simulink model "Copy_of_Qrotor_sim2"  (R2016a)
settings: Solver=ode4  StartTime=0.0  StopTime=T  FixedStep=0.001  RelTol=1e-3
values from neighbouring files (symbols this model uses):
  g = 9.81    [Sim_params.m]
  Ixx = 0.002100    (= 0.0021)    [Drone_params.m]
  Iyy = 0.002417    [Drone_params.m]
  Izz = 0.004633    [Drone_params.m]
  k_learn = 0.000001    (= 1e-06)    [Control_params.m]
  Ki = 3    [Control_params.m]
  KM_1 = KM_GENERAL    (= 0.00509)    [Drone_params.m]
  KM_2 = KM_GENERAL    (= 0.00509)    [Drone_params.m]
  KM_3 = KM_GENERAL    (= 0.00509)    [Drone_params.m]
  KM_4 = KM_GENERAL    (= 0.00509)    [Drone_params.m]
  KM_GENERAL = 0.00509    [Drone_params.m]
  KM_T_1 = KM_T_GENERAL    (= 5e-06)    [Drone_params.m]
  KM_T_2 = KM_T_GENERAL    (= 5e-06)    [Drone_params.m]
  KM_T_3 = KM_T_GENERAL    (= 5e-06)    [Drone_params.m]
  KM_T_4 = KM_T_GENERAL    (= 5e-06)    [Drone_params.m]
  KM_T_GENERAL = 0.000005    (= 5e-06)    [Drone_params.m]
  Kp = Ixx * Ki    [Control_params.m]
  KpP = 5    [Control_params.m]
  m = 0.475    [Drone_params.m]
  n_freq = 0.5    [Sim_params.m]
  PWM_CUT = 1000    [Drone_params.m]
  Tau_1 = Tau    (= 0.1)    [Drone_params.m]
  Tau_2 = Tau    (= 0.1)    [Drone_params.m]
  Tau_3 = Tau    (= 0.1)    [Drone_params.m]
  Tau_4 = Tau    (= 0.1)    [Drone_params.m]
  wnd_amp_p = .1    (= 0.1)    [Wind_params.m]
  wnd_amp_q = 0    [Wind_params.m]
  wnd_amp_r = 0    [Wind_params.m]
  wnd_amp_x = .1    (= 0.1)    [Wind_params.m]
  wnd_amp_y = .1    (= 0.1)    [Wind_params.m]
  wnd_amp_z = .1    (= 0.1)    [Wind_params.m]
  wnd_end_p = 20    [Wind_params.m]
  wnd_end_q = 15    [Wind_params.m]
  wnd_end_r = 15    [Wind_params.m]
  wnd_end_x = 44    [Wind_params.m]
  wnd_end_y = 31    [Wind_params.m]
  wnd_end_z = 49    [Wind_params.m]
  wnd_pqr_enable = 0    [Sim_params.m]
  wnd_ramp_p = 2*pi    (= 6.28318530718)    [Wind_params.m]
  wnd_ramp_q = 0.2    [Wind_params.m]
  wnd_ramp_r = 0.2    [Wind_params.m]
  wnd_ramp_x = .3    (= 0.3)    [Wind_params.m]
  wnd_ramp_y = .3    (= 0.3)    [Wind_params.m]
  wnd_ramp_z = .3    (= 0.3)    [Wind_params.m]
  wnd_start_p = 2    [Wind_params.m]
  wnd_start_q = 2    [Wind_params.m]
  wnd_start_r = 2    [Wind_params.m]
  wnd_start_x = 8    [Wind_params.m]
  wnd_start_y = 3    [Wind_params.m]
  wnd_start_z = 11    [Wind_params.m]
  wnd_xyz_enable = 0    [Sim_params.m]
  X_length = 0.155    [Drone_params.m]
  Y_length = 0.200    (= 0.2)    [Drone_params.m]
undefined symbols (not defined in the file or in its folder): X, Y, Z
libraries: simulink x12, sm_lib x10, nesl_utility x10
(part 2 of 2)

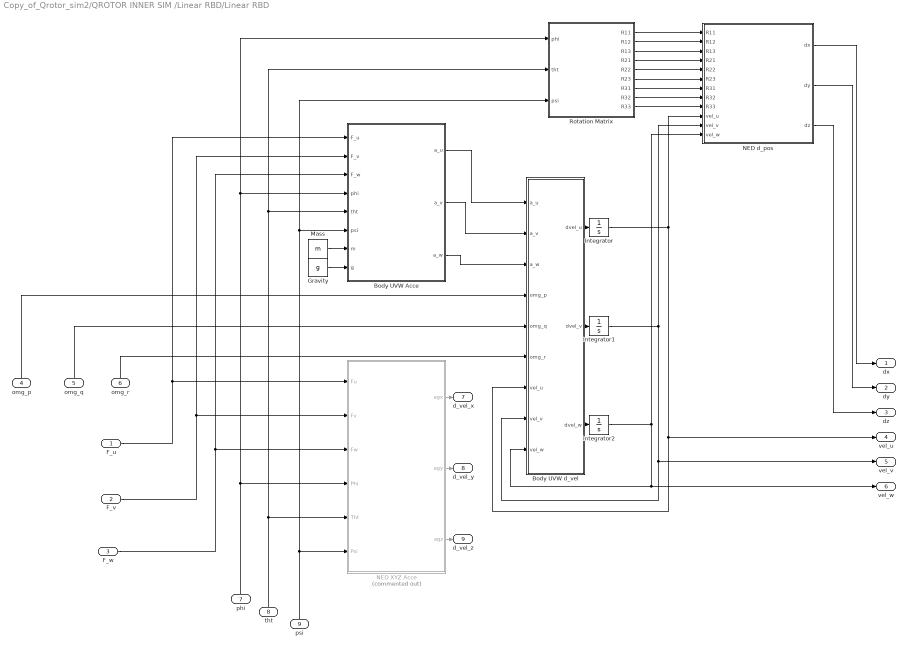
== system Copy_of_Qrotor_sim2/QROTOR INNER SIM /Linear RBD/Linear RBD ==
  F_u : Inport
  F_v : Inport  Port=2
  F_w : Inport  Port=3
  omg_p : Inport  Port=4
  omg_q : Inport  Port=5
  omg_r : Inport  Port=6
  phi : Inport  Port=7
  tht : Inport  Port=8
  psi : Inport  Port=9
  Body UVW Acce : MATLAB Function  TreatAsAtomicUnit=on
  Body UVW d_vel : MATLAB Function  TreatAsAtomicUnit=on
  Gravity : Constant  Value=g
  Integrator : Integrator
  Integrator1 : Integrator
  Integrator2 : Integrator
  Mass : Constant  Value=m
  NED XYZ Acce : Subsystem  Commented=on
  NED d_pos : MATLAB Function  TreatAsAtomicUnit=on
  Rotation Matrix : MATLAB Function  TreatAsAtomicUnit=on
  dx : Outport
  dy : Outport  Port=2
  dz : Outport  Port=3
  vel_u : Outport  Port=4
  vel_v : Outport  Port=5
  vel_w : Outport  Port=6
  d_vel_x : Outport  Port=7
  d_vel_y : Outport  Port=8
  "d_vel_z " : Outport  Port=9
  wires:
  NED d_pos/2(dy) -> dy/1
  Rotation Matrix/5(R22) -> NED d_pos/5(R22)
  NED d_pos/1(dx) -> dx/1
  F_v/1 -> Body UVW Acce/2(F_v), NED XYZ Acce/2(Fv)
  Mass/1 -> Body UVW Acce/7(m)
  Rotation Matrix/1(R11) -> NED d_pos/1(R11)
  Rotation Matrix/9(R33) -> NED d_pos/9(R33)
  Rotation Matrix/2(R12) -> NED d_pos/2(R12)
  Rotation Matrix/4(R21) -> NED d_pos/4(R21)
  F_w/1 -> Body UVW Acce/3(F_w), NED XYZ Acce/3(Fw)
  Rotation Matrix/6(R23) -> NED d_pos/6(R23)
  Rotation Matrix/7(R31) -> NED d_pos/7(R31)
  Rotation Matrix/8(R32) -> NED d_pos/8(R32)
  Gravity/1 -> Body UVW Acce/8(g)
  Rotation Matrix/3(R13) -> NED d_pos/3(R13)
  NED d_pos/3(dz) -> dz/1
  F_u/1 -> Body UVW Acce/1(F_u), NED XYZ Acce/1(Fu)
  Body UVW d_vel/3(dvel_w) -> Integrator2/1
  Body UVW d_vel/2(dvel_v) -> Integrator1/1
  Body UVW d_vel/1(dvel_u) -> Integrator/1
  NED XYZ Acce/1(agx) -> d_vel_x/1
  NED XYZ Acce/3(agz) -> "d_vel_z "/1
  omg_r/1 -> Body UVW d_vel/6(omg_r)
  NED XYZ Acce/2(agy) -> d_vel_y/1
  psi/1 -> Rotation Matrix/3(psi), Body UVW Acce/6(psi), NED XYZ Acce/6(Psi)
  tht/1 -> NED XYZ Acce/5(Tht), Body UVW Acce/5(tht), Rotation Matrix/2(tht)
  omg_q/1 -> Body UVW d_vel/5(omg_q)
  omg_p/1 -> Body UVW d_vel/4(omg_p)
  phi/1 -> NED XYZ Acce/4(Phi), Body UVW Acce/4(phi), Rotation Matrix/1(phi)
  Integrator/1 -> vel_u/1, Body UVW d_vel/7(vel_u), NED d_pos/10(vel_u)
  Integrator1/1 -> vel_v/1, Body UVW d_vel/8(vel_v), NED d_pos/11(vel_v)
  Integrator2/1 -> vel_w/1, Body UVW d_vel/9(vel_w), NED d_pos/12(vel_w)
  Body UVW Acce/2(a_v) -> Body UVW d_vel/2(a_v)
  Body UVW Acce/3(a_w) -> Body UVW d_vel/3(a_w)
  Body UVW Acce/1(a_u) -> Body UVW d_vel/1(a_u)

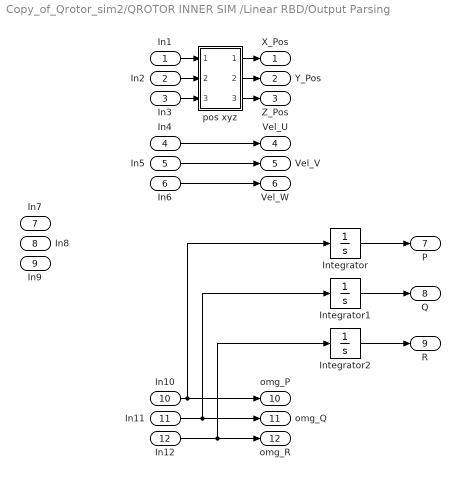
== system Copy_of_Qrotor_sim2/QROTOR INNER SIM /Linear RBD/Output Parsing ==
  In1 : Inport
  In2 : Inport  Port=2
  In3 : Inport  Port=3
  In4 : Inport  Port=4
  In5 : Inport  Port=5
  In6 : Inport  Port=6
  In7 : Inport  Port=7
  In8 : Inport  Port=8
  In9 : Inport  Port=9
  In10 : Inport  Port=10
  In11 : Inport  Port=11
  In12 : Inport  Port=12
  Integrator : Integrator
  Integrator1 : Integrator
  Integrator2 : Integrator
  pos xyz : Subsystem
  X_Pos : Outport
  Y_Pos : Outport  Port=2
  Z_Pos : Outport  Port=3
  Vel_U : Outport  Port=4
  Vel_V : Outport  Port=5
  Vel_W : Outport  Port=6
  P : Outport  Port=7
  Q : Outport  Port=8
  R : Outport  Port=9
  omg_P : Outport  Port=10
  omg_Q : Outport  Port=11
  omg_R : Outport  Port=12
  wires:
  In1/1 -> pos xyz/1(In1)
  pos xyz/2(Out2) -> Y_Pos/1
  pos xyz/1(Out1) -> X_Pos/1
  In2/1 -> pos xyz/2(In2)
  pos xyz/3(Out3) -> Z_Pos/1
  In3/1 -> pos xyz/3(In3)
  In10/1 -> Integrator/1, omg_P/1
  In11/1 -> Integrator1/1, omg_Q/1
  In6/1 -> Vel_W/1
  In5/1 -> Vel_V/1
  In4/1 -> Vel_U/1
  Integrator/1 -> P/1
  Integrator1/1 -> Q/1
  Integrator2/1 -> R/1
  In12/1 -> Integrator2/1, omg_R/1

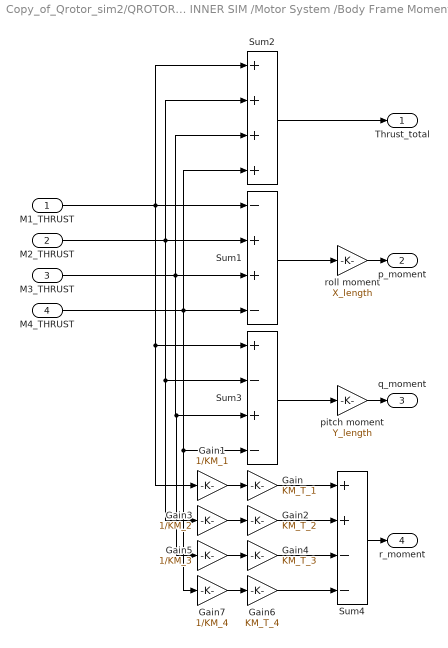
== system Copy_of_Qrotor_sim2/QROTOR INNER SIM /Motor System /Body Frame Moments ==
  M1_THRUST : Inport
  M2_THRUST : Inport  Port=2
  M3_THRUST : Inport  Port=3
  M4_THRUST : Inport  Port=4
  Gain : Gain  Gain=KM_T_1
  Gain1 : Gain  Gain=1/KM_1
  Gain2 : Gain  Gain=KM_T_2
  Gain3 : Gain  Gain=1/KM_2
  Gain4 : Gain  Gain=KM_T_3
  Gain5 : Gain  Gain=1/KM_3
  Gain6 : Gain  Gain=KM_T_4
  Gain7 : Gain  Gain=1/KM_4
  Sum1 : Sum  Inputs=-++-
  Sum2 : Sum  Inputs=++++
  Sum3 : Sum  Inputs=+-+-
  Sum4 : Sum  Inputs=++--
  pitch moment : Gain  Gain=Y_length
  roll moment : Gain  Gain=X_length
  Thrust_total : Outport
  p_moment : Outport  Port=2
  q_moment : Outport  Port=3
  "r_moment " : Outport  Port=4
  wires:
  Gain1/1 -> Gain/1
  Gain5/1 -> Gain4/1
  Gain7/1 -> Gain6/1
  Gain3/1 -> Gain2/1
  Gain2/1 -> Sum4/2
  Gain/1 -> Sum4/1
  Gain4/1 -> Sum4/3
  Gain6/1 -> Sum4/4
  M4_THRUST/1 -> Gain7/1, Sum3/4, Sum1/4, Sum2/4
  M1_THRUST/1 -> Gain1/1, Sum3/1, Sum2/1, Sum1/1
  Sum3/1 -> pitch moment/1
  Sum2/1 -> Thrust_total/1
  pitch moment/1 -> q_moment/1
  Sum4/1 -> "r_moment "/1
  roll moment/1 -> p_moment/1
  Sum1/1 -> roll moment/1
  M2_THRUST/1 -> Sum3/2, Gain3/1, Sum2/2, Sum1/2
  M3_THRUST/1 -> Gain5/1, Sum3/3, Sum2/3, Sum1/3

== system Copy_of_Qrotor_sim2/QROTOR INNER SIM /Motor System /Command to Motor Map ==
  P_TORQUE : Inport
  Q_TORQUE : Inport  Port=2
  R_TORQUE : Inport  Port=3
  THRUST : Inport  Port=4
  Constant : Constant  Value=PWM_CUT
  Pitch : Gain  Gain=1/(4 * KM_GENERAL * Y_length)
  Roll : Gain  Gain=1/(4 * KM_GENERAL * X_length)
  Sum : Sum  Inputs=-++++
  Sum1 : Sum  Inputs=+-+++
  Sum2 : Sum  Inputs=++-++
  Sum3 : Sum  Inputs=---++
  Thrust : Gain  Gain=1/(4 * KM_GENERAL)
  Yaw : Gain  Gain=1/(4 * KM_T_GENERAL)
  M1_PWM : Outport
  M2_PWM : Outport  Port=2
  M3_PWM : Outport  Port=3
  M4_PWM : Outport  Port=4
  wires:
  Sum2/1 -> M3_PWM/1
  Sum3/1 -> M4_PWM/1
  R_TORQUE/1 -> Yaw/1
  THRUST/1 -> Thrust/1
  Sum/1 -> M1_PWM/1
  P_TORQUE/1 -> Roll/1
  Q_TORQUE/1 -> Pitch/1
  Sum1/1 -> M2_PWM/1
  Yaw/1 -> Sum2/3, Sum1/3, Sum/3, Sum3/3
  Thrust/1 -> Sum3/4, Sum2/4, Sum1/4, Sum/4
  Roll/1 -> Sum/1, Sum1/1, Sum2/1, Sum3/1
  Pitch/1 -> Sum/2, Sum1/2, Sum2/2, Sum3/2
  Constant/1 -> Sum3/5, Sum2/5, Sum1/5, Sum/5

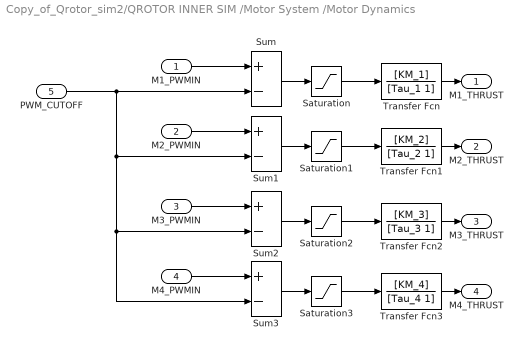
== system Copy_of_Qrotor_sim2/QROTOR INNER SIM /Motor System /Motor Dynamics ==
  M1_PWMIN : Inport
  M2_PWMIN : Inport  Port=2
  M3_PWMIN : Inport  Port=3
  M4_PWMIN : Inport  Port=4
  "PWM_CUTOFF " : Inport  Port=5
  Saturation{,1..3} (4 alike) : Saturate  UpperLimit=1000  LowerLimit=0
  Sum{,1..3} (4 alike) : Sum  Inputs=+-
  Transfer Fcn : TransferFcn  Numerator=[KM_1]  Denominator=[Tau_1 1]
  Transfer Fcn1 : TransferFcn  Numerator=[KM_2]  Denominator=[Tau_2 1]
  Transfer Fcn2 : TransferFcn  Numerator=[KM_3]  Denominator=[Tau_3 1]
  Transfer Fcn3 : TransferFcn  Numerator=[KM_4]  Denominator=[Tau_4 1]
  M1_THRUST : Outport
  M2_THRUST : Outport  Port=2
  M3_THRUST : Outport  Port=3
  M4_THRUST : Outport  Port=4
  wires:
  Transfer Fcn1/1 -> M2_THRUST/1
  Transfer Fcn/1 -> M1_THRUST/1
  Transfer Fcn2/1 -> M3_THRUST/1
  Transfer Fcn3/1 -> M4_THRUST/1
  Sum1/1 -> Saturation1/1
  M4_PWMIN/1 -> Sum3/1
  Sum3/1 -> Saturation3/1
  M3_PWMIN/1 -> Sum2/1
  Sum2/1 -> Saturation2/1
  M2_PWMIN/1 -> Sum1/1
  M1_PWMIN/1 -> Sum/1
  Sum/1 -> Saturation/1
  "PWM_CUTOFF "/1 -> Sum3/2, Sum2/2, Sum1/2, Sum/2
  Saturation/1 -> Transfer Fcn/1
  Saturation1/1 -> Transfer Fcn1/1
  Saturation2/1 -> Transfer Fcn2/1
  Saturation3/1 -> Transfer Fcn3/1

== system Copy_of_Qrotor_sim2/QROTOR INNER SIM /Linear RBD/Linear RBD/NED XYZ Acce ==
  Fu : Inport
  Fv : Inport  Port=2
  Fw : Inport  Port=3
  Phi : Inport  Port=4
  Tht : Inport  Port=5
  Psi : Inport  Port=6
  Acceleration X : MATLAB Function  TreatAsAtomicUnit=on
  Acceleration Y : MATLAB Function  TreatAsAtomicUnit=on
  Acceleration Z : MATLAB Function  TreatAsAtomicUnit=on
  Gravity : Constant  Value=g
  Mass : Constant  Value=m
  Rotation Matrix : MATLAB Function  TreatAsAtomicUnit=on
  agx : Outport
  agy : Outport  Port=2
  agz : Outport  Port=3
  wires:
  Rotation Matrix/6(R23) -> Acceleration Y/3(R23)
  Rotation Matrix/7(R31) -> Acceleration Z/1(R31)
  Rotation Matrix/1(R11) -> Acceleration X/1(R11)
  Rotation Matrix/2(R12) -> Acceleration X/2(R12)
  Fv/1 -> Acceleration Z/5(F_v), Acceleration Y/5(F_v), Acceleration X/5(F_v)
  Fw/1 -> Acceleration Z/6(F_w), Acceleration Y/6(F_w), Acceleration X/6(F_w)
  Rotation Matrix/3(R13) -> Acceleration X/3(R13)
  Rotation Matrix/4(R21) -> Acceleration Y/1(R21)
  Rotation Matrix/5(R22) -> Acceleration Y/2(R22)
  Rotation Matrix/9(R33) -> Acceleration Z/3(R33)
  Rotation Matrix/8(R32) -> Acceleration Z/2(R32)
  Acceleration Z/1(agz) -> agz/1
  Acceleration Y/1(agy) -> agy/1
  Psi/1 -> Rotation Matrix/3(psi)
  Phi/1 -> Rotation Matrix/1(phi)
  Acceleration X/1(agx) -> agx/1
  Mass/1 -> Acceleration Y/7(m), Acceleration X/7(m), Acceleration Z/7(m)
  Tht/1 -> Rotation Matrix/2(tht)
  Fu/1 -> Acceleration Z/4(F_u), Acceleration Y/4(F_u), Acceleration X/4(F_u)
  Gravity/1 -> Acceleration Z/8(g)

== system Copy_of_Qrotor_sim2/QROTOR INNER SIM /Linear RBD/Output Parsing/pos xyz ==
  In1 : Inport
  In2 : Inport  Port=2
  In3 : Inport  Port=3
  Integrator6 : Integrator
  Integrator7 : Integrator
  Integrator8 : Integrator
  Out1 : Outport
  Out2 : Outport  Port=2
  Out3 : Outport  Port=3
  wires:
  In3/1 -> Integrator8/1
  In1/1 -> Integrator6/1
  In2/1 -> Integrator7/1
  Integrator6/1 -> Out1/1
  Integrator8/1 -> Out3/1
  Integrator7/1 -> Out2/1

== matlab function Copy_of_Qrotor_sim2/QROTOR INNER SIM /Linear RBD/Linear RBD/NED XYZ Acce/Rotation Matrix ==
  data: phi input; R11 output; tht input; psi input; R12 output; R13 output; R21 output; R22 output; R23 output; R31 output; R32 output; R33 output
function [R11, R12, R13, R21, R22, R23, R31, R32, R33] = fcn(phi, tht, psi)

R11 = cos(psi)*cos(tht);
R12 = cos(psi)*sin(tht)*sin(phi) - sin(psi)*cos(phi);
R13 = cos(psi)*sin(tht)*cos(phi) + sin(psi)*sin(phi);
R21 = sin(psi)*cos(tht);
R22 = sin(psi)*sin(tht)*sin(phi) + cos(psi)*cos(phi);
R23 = sin(psi)*sin(tht)*cos(phi) - cos(psi)*sin(phi);
R31 = -sin(tht);
R32 = cos(tht)*sin(phi);
R33 = cos(tht)*cos(phi);

end

== matlab function Copy_of_Qrotor_sim2/QROTOR INNER SIM /Angular RBD/RBD Angular Rate ==
  data: omg_p input; phi_dot output; omg_q input; omg_r input; phi input; tht input; psi input; tht_dot output; psi_dot output
function [phi_dot, tht_dot, psi_dot] = fcn(omg_p, omg_q, omg_r, phi, tht, psi)

phi_dot = [1  sin(phi)*tan(tht)  cos(phi)*tan(tht)] * [omg_p; omg_q; omg_r];
tht_dot = [0       cos(phi)          -sin(phi)    ] * [omg_p; omg_q; omg_r];
psi_dot = [0  sin(phi)*sec(tht)  cos(phi)*sec(tht)] * [omg_p; omg_q; omg_r];

end

== matlab function Copy_of_Qrotor_sim2/QROTOR INNER SIM /Linear RBD/Linear RBD/NED XYZ Acce/Acceleration X ==
  data: R11 input; agx output; R12 input; R13 input; F_u input; F_v input; F_w input; m input
function agx = fcn(R11, R12, R13, F_u, F_v, F_w, m)

agx = [R11 R12 R13] * [ F_u; F_v; F_w; ] / m;

end

== matlab function Copy_of_Qrotor_sim2/QROTOR INNER SIM /Linear RBD/Linear RBD/NED XYZ Acce/Acceleration Y ==
  data: R21 input; agy output; R22 input; R23 input; F_u input; F_v input; F_w input; m input
function agy = fcn(R21, R22, R23, F_u, F_v, F_w, m)

agy = [R21 R22 R23] * [ F_u; F_v; F_w; ] / m;

end

== matlab function Copy_of_Qrotor_sim2/QROTOR INNER SIM /Linear RBD/Linear RBD/NED XYZ Acce/Acceleration Z ==
  data: R31 input; agz output; R32 input; R33 input; F_u input; F_v input; F_w input; m input; g input
function agz = fcn(R31, R32, R33, F_u, F_v, F_w, m, g)

agz = [R31 R32 R33] * [ F_u; F_v; F_w; ] / m + g;

end

== matlab function Copy_of_Qrotor_sim2/QROTOR INNER SIM /Linear RBD/Linear RBD/Body UVW Acce ==
  data: F_u input; F_v input; F_w input; phi input; tht input; psi input; m input; a_u output; g input; a_v output; a_w output
function [a_u, a_v, a_w] = fcn(F_u, F_v, F_w, phi, tht, psi, m, g)

a_u = F_u / m - g * sin(tht);
a_v = F_v / m + g * sin(phi)*cos(tht);
a_w = F_w / m + g * cos(phi)*cos(tht);

end

== matlab function Copy_of_Qrotor_sim2/QROTOR INNER SIM /Linear RBD/Linear RBD/Body UVW d_vel ==
  data: a_u input; dvel_u output; a_v input; a_w input; omg_p input; omg_q input; omg_r input; vel_u input; vel_v input; vel_w input; dvel_v output; dvel_w output
function [dvel_u, dvel_v, dvel_w] = fcn(a_u, a_v, a_w, omg_p, omg_q, omg_r, vel_u, vel_v, vel_w)

dvel_u = a_u - omg_q*vel_w + omg_r*vel_v;
dvel_v = a_v - omg_r*vel_u + omg_p*vel_w;
dvel_w = a_w - omg_p*vel_v + omg_q*vel_u;

end

== matlab function Copy_of_Qrotor_sim2/QROTOR INNER SIM /Linear RBD/Linear RBD/Rotation Matrix ==
  data: phi input; R11 output; tht input; psi input; R12 output; R13 output; R21 output; R22 output; R23 output; R31 output; R32 output; R33 output
function [R11, R12, R13, R21, R22, R23, R31, R32, R33] = fcn(phi, tht, psi)

R11 = cos(psi)*cos(tht);
R12 = cos(psi)*sin(tht)*sin(phi) - sin(psi)*cos(phi);
R13 = cos(psi)*sin(tht)*cos(phi) + sin(psi)*sin(phi);
R21 = sin(psi)*cos(tht);
R22 = sin(psi)*sin(tht)*sin(phi) + cos(psi)*cos(phi);
R23 = sin(psi)*sin(tht)*cos(phi) - cos(psi)*sin(phi);
R31 = -sin(tht);
R32 = cos(tht)*sin(phi);
R33 = cos(tht)*cos(phi);

end

== matlab function Copy_of_Qrotor_sim2/QROTOR INNER SIM /Linear RBD/Linear RBD/NED d_pos ==
  data: R11 input; dx output; R12 input; R13 input; R21 input; R22 input; R23 input; R31 input; R32 input; R33 input; vel_u input; vel_v input; vel_w input; dy output; dz output
function [dx,dy,dz] = fcn(R11, R12, R13, R21, R22, R23, R31, R32, R33, vel_u, vel_v, vel_w)

R = [ R11 R12 R13;
      R21 R22 R23;
      R31 R32 R33 ];

dpos = R * [vel_u; vel_v; vel_w];

dx = dpos(1);
dy = dpos(2);
dz = dpos(3);

end

== matlab function Copy_of_Qrotor_sim2/QROTOR INNER SIM /Angular RBD/RBD Angular Acce/AngularRBD_AcceCalc ==
  data: M_p input; domg_p output; M_q input; M_r input; omg_p input; omg_q input; omg_r input; domg_q output; domg_r output; Ixx input; Iyy input; Izz input
function [domg_p, domg_q, domg_r] = fcn(M_p, M_q, M_r, omg_p, omg_q, omg_r, Ixx, Iyy, Izz)

domg_p = ( ( Iyy - Izz ) * omg_q * omg_r + M_p ) / Ixx; 
domg_q = ( ( Ixx - Izz ) * omg_p * omg_r + M_q ) / Iyy;
domg_r = ( ( Ixx - Iyy ) * omg_p * omg_q + M_r ) / Izz;

end

== matlab function Copy_of_Qrotor_sim2/Subsystem/Iym Predictor ==
  data: domg_P input; p_torque input; Iym_sim_out output; k_learn input; Iym_sim input
function Iym_sim_out = fcn(domg_P, p_torque, k_learn, Iym_sim)

e = abs(domg_P - p_torque) / Iym_sim;
Iym_sim_out = Iym_sim - k_learn * e;

end

== matlab function Copy_of_Qrotor_sim2/Subsystem1/Ixm Predictor ==
  data: domg_P input; p_torque input; Ixm_sim_out output; k_learn input; Ixm_sim input
function Ixm_sim_out = fcn(domg_P, p_torque, k_learn, Ixm_sim)

e = abs(domg_P - p_torque) / Ixm_sim;
Ixm_sim_out = Ixm_sim - k_learn * e;

end
